simulink model "BD_FUZZY_EMISSIONS"  (Simulink 4.1.1)
settings: Solver=ode1  SolverMode=SingleTasking  StartTime=0.0  StopTime=max(cyc_mph(:,1))  FixedStep=1  MaxStep=1  RelTol=1e-3  AbsTol=1e-3
undefined symbols (not defined in the file): cs_hi_soc, cs_lo_soc, ex_calc, fc_emis, fc_map_spd, fc_max_trq, fc_spd_scale, fc_trq_scale, fc_tstat, fuzzy_target_compute_emissions, mfuzzy_emissions, vc_fc_warm_tmp_frac
libraries: lib_transmission x4, lib_wheel x2, lib_help x2, lib_outputs x1, lib_controls x1, lib_interactive x1, lib_drive_cycle x1, lib_energy_storage x1, lib_exhaust x1, lib_fuel_converter x1, lib_electric_machine x1, lib_power_bus x1
settings Model: LastModifiedBy=ssprik  ModifiedComment=ssprik -- Wed Sep 24 14:56:58 2003 -- Version 1.295  SaveTime=off  SaveOutput=off  LimitDataPoints=off  UnconnectedLineMsg=none  RTWTemplateMakefile=grt_vc.tmf  ExtModeTrigMode=oneshot  ExtModeArmWhenConnect=off
settings Model: ModifiedHistory=|
  | ssprik -- Wed Sep 24 14:56:58 2003 -- Version 1.295
  | 
  | 
  | abrooker -- Tue May 14 11:44:18 2002 -- Version 1.294
  | 
  | 
  | mokeefe -- Thu Apr 18 07:56:06 2002 -- Version 1.293
  | saving the model:
  | o "without the model browser open"
  | o with only top-level screen visible
  | o and with "fit to view" enabled
  | 
  | mokeefe -- Thu Apr 18 07:46:20 2002 -- Version 1.292
  | saving the model:
  | o "without the model browser open"
  | o with only top-level screen visible
  | o and with "fit to view" enabled

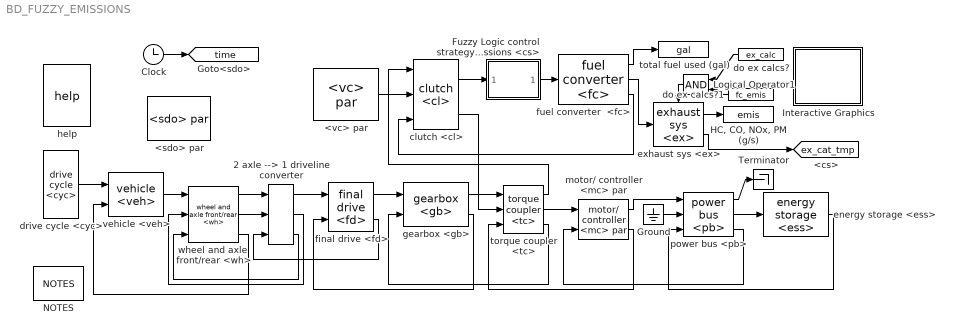
== system BD_FUZZY_EMISSIONS ==
  2 axle --> 1 driveline converter : lib_wheel/2 axle --> 1 driveline converter
      settings: RTWFcnNameOpts=Auto  RTWFileNameOpts=Auto
  <sdo> par : lib_outputs/<sdo> par
  <vc> par : lib_controls/<vc> par
  Clock : Clock
      settings: DisplayTime=off  Decimation=10
  Fuzzy Logic control strategy with Emissions <cs> : Subsystem
      settings: RTWFcnNameOpts=Auto  RTWFileNameOpts=Auto
      mask Display: image(imread('bdi_fuzzy.jpg'))
  Ground : Ground
  "HC, CO, NOx, PM (g/s)" : ToWorkspace  VariableName=emis  SampleTime=0  SaveFormat=Array
  Interactive Graphics : Subsystem  BlockChoice=off
      settings: AttributesFormatString=%<BlockChoice>  TemplateBlock=lib_interactive/Interactive Graphics  MemberBlocks=off,on  RTWFcnNameOpts=Auto  RTWFileNameOpts=Auto
  Logical Operator1 : Logic  Orientation=left  Operator=AND  Inputs=2
  NOTES : lib_help/NOTES
  Terminator : Terminator
  clutch <cl> : lib_transmission/clutch <cl>  slip_spd=vc_launch_spd  maxtrq=max(fc_max_trq)*fc_trq_scale
  do ex calcs? : Constant  Orientation=left  Value=ex_calc
  do ex calcs?1 : Constant  Orientation=left  Value=fc_emis
  drive cycle <cyc> : lib_drive_cycle/drive cycle <cyc>
  energy storage <ess> : lib_energy_storage/energy storage <ess>  AncestorBlock=lib_energy_storage/Subsystem/energy storage <ess>
  exhaust sys <ex> : lib_exhaust/exhaust sys <ex>
  final drive <fd> : lib_transmission/final drive <fd>
  fuel converter  <fc> : lib_fuel_converter/fuel converter  <fc>
  gearbox <gb> : lib_transmission/gearbox <gb>
  help : lib_help/help
  motor/ controller <mc> par : lib_electric_machine/motor// controller <mc> par
  power bus <pb> : lib_power_bus/power bus <pb>
  torque coupler <tc> : lib_transmission/torque coupler <tc>
  total fuel used (gal) : ToWorkspace  VariableName=gal  SampleTime=0  SaveFormat=Array
  vehicle <veh> : lib_vehicle/vehicle <veh>
  wheel and axle  front/rear <wh> : lib_wheel/wheel and axle  front//rear <wh>
  tag scope: ex_cat_tmp=global, time=global
  wires:
  wheel and axle  front/rear <wh>/3 -> vehicle <veh>/2
  final drive <fd>/1 -> gearbox <gb>/1
  drive cycle <cyc>/1 -> vehicle <veh>/1
  clutch <cl>/1 -> Fuzzy Logic control strategy with Emissions <cs>/1("trq and spd req'd into clutch (N*m, rad/s)")
  Fuzzy Logic control strategy with Emissions <cs>/1("trq and spd req'd from engine (N*m, rad/s)") -> fuel converter  <fc>/1
  fuel converter  <fc>/2 -> exhaust sys <ex>/1
  do ex calcs?/1 -> Logical Operator1/1
  fuel converter  <fc>/3 -> clutch <cl>/3
  fuel converter  <fc>/1 -> total fuel used (gal)/1
  exhaust sys <ex>/1 -> "HC, CO, NOx, PM (g/s)"/1
  Logical Operator1/1 -> exhaust sys <ex>/Enable
  do ex calcs?1/1 -> Logical Operator1/2
  Clock/1 -> [time]
  gearbox <gb>/2 -> final drive <fd>/2
  torque coupler <tc>/3 -> gearbox <gb>/2
  torque coupler <tc>/1 -> clutch <cl>/1
  clutch <cl>/2 -> torque coupler <tc>/2
  gearbox <gb>/1 -> torque coupler <tc>/1
  <vc> par/1 -> clutch <cl>/2
  motor/ controller <mc> par/2 -> torque coupler <tc>/3
  motor/ controller <mc> par/1 -> power bus <pb>/1
  Ground/1 -> power bus <pb>/2
  power bus <pb>/3 -> motor/ controller <mc> par/2
  power bus <pb>/2 -> energy storage <ess>/1
  power bus <pb>/1 -> Terminator/1
  energy storage <ess>/1 -> power bus <pb>/3
  torque coupler <tc>/2 -> motor/ controller <mc> par/1
  exhaust sys <ex>/2 -> [ex_cat_tmp]
  vehicle <veh>/1 -> wheel and axle  front/rear <wh>/1
  wheel and axle  front/rear <wh>/1 -> 2 axle --> 1 driveline converter/1
  wheel and axle  front/rear <wh>/2 -> 2 axle --> 1 driveline converter/2
  2 axle --> 1 driveline converter/1 -> final drive <fd>/1
  2 axle --> 1 driveline converter/2 -> wheel and axle  front/rear <wh>/2
  2 axle --> 1 driveline converter/3 -> wheel and axle  front/rear <wh>/3
  final drive <fd>/2 -> 2 axle --> 1 driveline converter/3

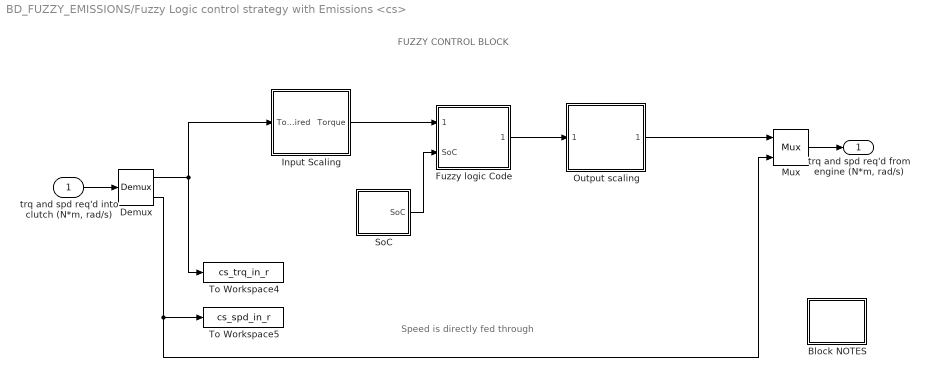
== system BD_FUZZY_EMISSIONS/Fuzzy Logic control strategy with Emissions <cs> ==
  note: FUZZY CONTROL BLOCK
  note: Speed is directly fed through
  "trq and spd req'd into clutch (N*m, rad/s)" : Inport  Port=1  LatchInput=off
  Block NOTES : Subsystem
      settings: RTWFcnNameOpts=Auto  RTWFileNameOpts=Auto
      mask Display: disp('Block\nNOTES')
  Demux : Demux  Outputs=2  BusSelectionMode=off
  Fuzzy logic Code : Subsystem
      settings: RTWFcnNameOpts=Auto  RTWFileNameOpts=Auto
  Input Scaling : Subsystem
      settings: RTWFcnNameOpts=Auto  RTWFileNameOpts=Auto
  Mux : Mux  Inputs=2
      settings: DisplayOption=none
  Output scaling : Subsystem
      settings: RTWFcnNameOpts=Auto  RTWFileNameOpts=Auto
  "SoC " : Subsystem
      settings: RTWFcnNameOpts=Auto  RTWFileNameOpts=Auto
  To Workspace4 : ToWorkspace  VariableName=cs_trq_in_r  SampleTime=-1  SaveFormat=Array
  To Workspace5 : ToWorkspace  VariableName=cs_spd_in_r  SampleTime=-1  SaveFormat=Array
  "trq and spd req'd from engine (N*m, rad/s)" : Outport  Port=1
  wires:
  Fuzzy logic Code/1(delta  alpha) -> Output scaling/1("delta alpha ")
  Input Scaling/1(Torque) -> Fuzzy logic Code/1(Torque)
  "trq and spd req'd into clutch (N*m, rad/s)"/1 -> Demux/1
  Demux/2 -> To Workspace5/1, Mux/2
  Demux/1 -> To Workspace4/1, Input Scaling/1(Torque required)
  Mux/1 -> "trq and spd req'd from engine (N*m, rad/s)"/1
  "SoC "/1(SoC) -> Fuzzy logic Code/2(SoC)
  Output scaling/1(ICE Torque command) -> Mux/1

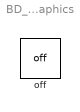
== system BD_FUZZY_EMISSIONS/Interactive Graphics ==
  off : lib_interactive/off  Tag=Altia_off  Orientation=up

== system BD_FUZZY_EMISSIONS/Fuzzy Logic control strategy with Emissions <cs>/Block NOTES ==
  note: The Fuzzy Control Block takes in the torque and speed requested by the clutch (sink) and calculates
      | the torque split between the ICE and the Motor. The fuzzy logic algorithm sets a base (optimal)
      | operating point of the ICE and modifies the actual operating point about the optimal, based on
      | the actual torque request and the battery State of Charge (SOC). Finally, a torque request is sent to the
      | ICE and the motor buffers the remaining torque (positive or negative).

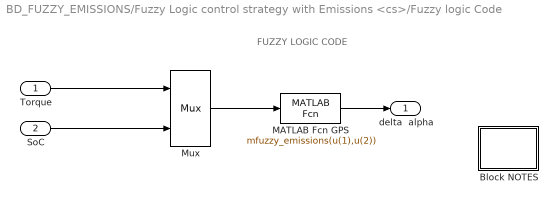
== system BD_FUZZY_EMISSIONS/Fuzzy Logic control strategy with Emissions <cs>/Fuzzy logic Code ==
  note: FUZZY LOGIC CODE
  Torque : Inport  Port=1  LatchInput=off
  SoC : Inport  Port=2  LatchInput=off
  Block NOTES : Subsystem
      settings: RTWFcnNameOpts=Auto  RTWFileNameOpts=Auto
      mask Display: disp('Block\nNOTES')
  "MATLAB Fcn GPS " : MATLABFcn  MATLABFcn=mfuzzy_emissions(u(1),u(2))  OutputDimensions=1  OutputSignalType=auto  Output1D=on
  Mux : Mux  Inputs=2
      settings: DisplayOption=none
  delta  alpha : Outport  Port=1
  wires:
  Mux/1 -> "MATLAB Fcn GPS "/1
  Torque/1 -> Mux/1
  "MATLAB Fcn GPS "/1 -> delta  alpha/1
  SoC/1 -> Mux/2

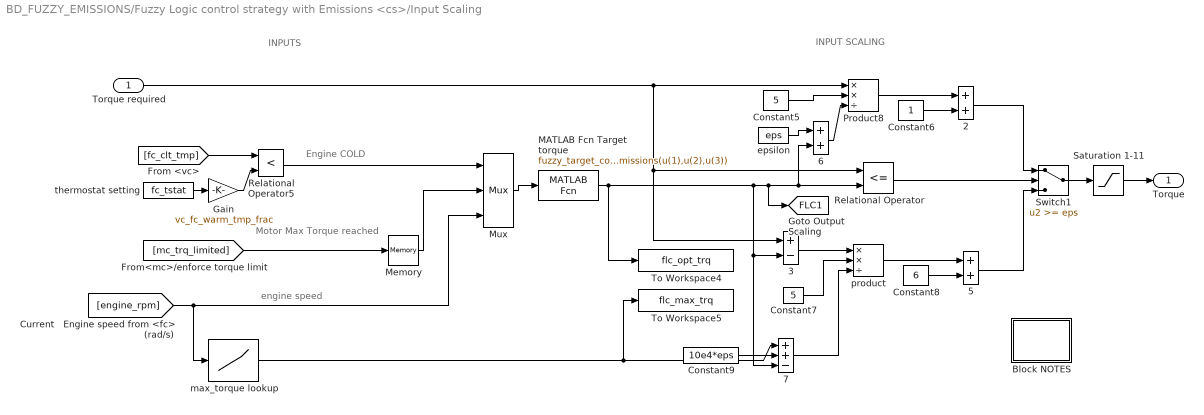
== system BD_FUZZY_EMISSIONS/Fuzzy Logic control strategy with Emissions <cs>/Input Scaling ==
  note: INPUTS
  note: INPUT SCALING
  note: Engine COLD
  note: Motor Max
      | Torque reached
  note: engine speed
  Torque required : Inport  Port=1  LatchInput=off
  " 2" : Sum  Inputs=++  SaturateOnIntegerOverflow=on
  " 3" : Sum  Inputs=+-  SaturateOnIntegerOverflow=on
  " 5" : Sum  Inputs=++  SaturateOnIntegerOverflow=on
  " 6" : Sum  Inputs=++  SaturateOnIntegerOverflow=on
  " 7" : Sum  Inputs=++-  SaturateOnIntegerOverflow=on
  Block NOTES : Subsystem
      settings: RTWFcnNameOpts=Auto  RTWFileNameOpts=Auto
      mask Display: disp('Block\nNOTES')
  Constant5 : Constant  Value=5
  Constant6 : Constant  Value=1
  Constant7 : Constant  Value=5
  Constant8 : Constant  Value=6
  Constant9 : Constant  Value=10e4*eps
  Gain : Gain  Gain=vc_fc_warm_tmp_frac  Multiplication=Element-wise(K.*u)  SaturateOnIntegerOverflow=on
  MATLAB Fcn Target torque : MATLABFcn  MATLABFcn=fuzzy_target_compute_emissions(u(1),u(2),u(3))  OutputDimensions=1  OutputSignalType=auto  Output1D=on
  Memory : Memory  X0=0  InheritSampleTime=off
      settings: RTWStateStorageClass=Auto
  Mux : Mux  Inputs=3
      settings: DisplayOption=none
  Product8 : Product  Inputs=**/  Multiplication=Element-wise(.*)  SaturateOnIntegerOverflow=on
  Relational Operator : RelationalOperator  Operator=<=
  Relational Operator5 : RelationalOperator  Operator=<
  "Saturation 1-11 " : Saturate  UpperLimit=11  LowerLimit=1  LinearizeAsGain=on
  Switch1 : Switch  Threshold=eps
  To Workspace4 : ToWorkspace  VariableName=flc_opt_trq  SampleTime=-1  SaveFormat=Array
  To Workspace5 : ToWorkspace  VariableName=flc_max_trq  SampleTime=-1  SaveFormat=Array
  epsilon : Constant  Value=eps
  max_torque lookup : Lookup  InputValues=fc_map_spd*fc_spd_scale  OutputValues=fc_max_trq*fc_trq_scale
  product : Product  Inputs=**/  Multiplication=Element-wise(.*)  SaturateOnIntegerOverflow=on
  thermostat setting : Constant  Value=fc_tstat
  Torque : Outport  Port=1
  tag scope: FLC1=global
  wires:
  Switch1/1 -> "Saturation 1-11 "/1
  " 7"/1 -> product/3
  " 6"/1 -> Product8/3
  epsilon/1 -> " 6"/1
  Constant9/1 -> " 7"/2
  Constant5/1 -> Product8/2
  "Saturation 1-11 "/1 -> Torque/1
  " 5"/1 -> Switch1/3
  product/1 -> " 5"/1
  Constant8/1 -> " 5"/2
  Constant7/1 -> product/2
  " 3"/1 -> product/1
  " 2"/1 -> Switch1/1
  Constant6/1 -> " 2"/2
  Product8/1 -> " 2"/1
  Relational Operator/1 -> Switch1/2
  MATLAB Fcn Target torque/1 -> To Workspace4/1, " 7"/3, " 3"/2, " 6"/2, Relational Operator/2, [FLC1]
  [engine_rpm] -> max_torque lookup/1, Mux/3
  Mux/1 -> MATLAB Fcn Target torque/1
  max_torque lookup/1 -> " 7"/1, To Workspace5/1
  Torque required/1 -> " 3"/1, Relational Operator/1, Product8/1
  [mc_trq_limited] -> Memory/1
  thermostat setting/1 -> Gain/1
  Gain/1 -> Relational Operator5/2
  [fc_clt_tmp] -> Relational Operator5/1
  Relational Operator5/1 -> Mux/1
  Memory/1 -> Mux/2

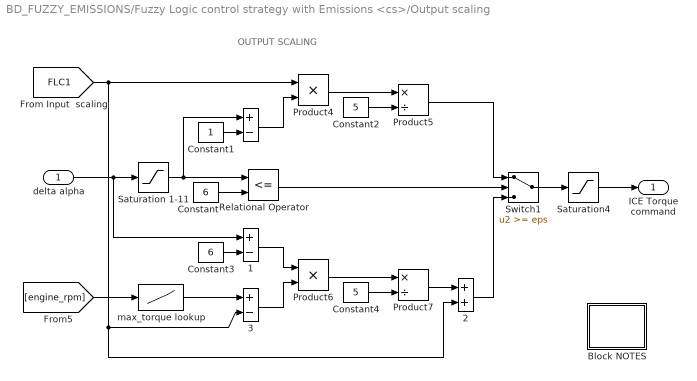
== system BD_FUZZY_EMISSIONS/Fuzzy Logic control strategy with Emissions <cs>/Output scaling ==
  note: OUTPUT SCALING
  "delta alpha " : Inport  Port=1  LatchInput=off
  " " : Sum  Inputs=+-  SaturateOnIntegerOverflow=on
  " 1" : Sum  Inputs=+-  SaturateOnIntegerOverflow=on
  " 2" : Sum  Inputs=++  SaturateOnIntegerOverflow=on
  " 3" : Sum  Inputs=+-  SaturateOnIntegerOverflow=on
  Block NOTES : Subsystem
      settings: RTWFcnNameOpts=Auto  RTWFileNameOpts=Auto
      mask Display: disp('Block\nNOTES')
  Constant : Constant  Value=6
  Constant1 : Constant  Value=1
  Constant2 : Constant  Value=5
  Constant3 : Constant  Value=6
  Constant4 : Constant  Value=5
  Product4 : Product  Inputs=2  Multiplication=Element-wise(.*)  SaturateOnIntegerOverflow=on
  Product5 : Product  Inputs=*/  Multiplication=Element-wise(.*)  SaturateOnIntegerOverflow=on
  Product6 : Product  Inputs=2  Multiplication=Element-wise(.*)  SaturateOnIntegerOverflow=on
  Product7 : Product  Inputs=*/  Multiplication=Element-wise(.*)  SaturateOnIntegerOverflow=on
  Relational Operator : RelationalOperator  Operator=<=
  Saturation 1-11 : Saturate  UpperLimit=11  LowerLimit=1  LinearizeAsGain=on
  Saturation4 : Saturate  UpperLimit=max(fc_max_trq*fc_trq_scale)  LowerLimit=0  LinearizeAsGain=on
  Switch1 : Switch  Threshold=eps
  max_torque lookup : Lookup  InputValues=fc_map_spd*fc_spd_scale  OutputValues=fc_max_trq*fc_trq_scale
  ICE Torque command : Outport  Port=1
  wires:
  max_torque lookup/1 -> " 3"/1
  [engine_rpm] -> max_torque lookup/1
  Saturation4/1 -> ICE Torque command/1
  Switch1/1 -> Saturation4/1
  Product7/1 -> " 2"/1
  " 2"/1 -> Switch1/3
  Relational Operator/1 -> Switch1/2
  Product5/1 -> Switch1/1
  Constant4/1 -> Product7/2
  Product6/1 -> Product7/1
  " 3"/1 -> Product6/2
  " 1"/1 -> Product6/1
  Constant3/1 -> " 1"/2
  "delta alpha "/1 -> Saturation 1-11/1, " 1"/1
  [FLC1] -> " 3"/2, " 2"/2, Product4/1
  Constant2/1 -> Product5/2
  Product4/1 -> Product5/1
  " "/1 -> Product4/2
  Saturation 1-11/1 -> " "/1, Relational Operator/1
  Constant1/1 -> " "/2
  Constant/1 -> Relational Operator/2

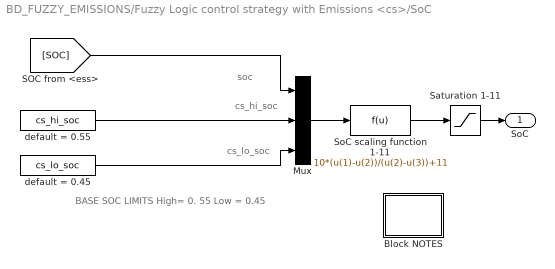
== system BD_FUZZY_EMISSIONS/Fuzzy Logic control strategy with Emissions <cs>/SoC  ==
  note: soc
  note: cs_hi_soc
  note: cs_lo_soc
  note: BASE SOC LIMITS
      | High= 0. 55
      | Low  = 0.45
  Block NOTES : Subsystem
      settings: RTWFcnNameOpts=Auto  RTWFileNameOpts=Auto
      mask Display: disp('Block\nNOTES')
  Mux : Mux  Inputs=3
  Saturation 1-11 : Saturate  UpperLimit=11  LowerLimit=1  LinearizeAsGain=on
  SoC scaling function 1-11 : Fcn  Expr=10*(u(1)-u(2))/(u(2)-u(3))+11
  default = 0.45 : Constant  Value=cs_lo_soc
  default = 0.55 : Constant  Value=cs_hi_soc
  SoC : Outport  Port=1
  wires:
  Mux/1 -> SoC scaling function 1-11/1
  [SOC] -> Mux/1
  default = 0.55/1 -> Mux/2
  default = 0.45/1 -> Mux/3
  SoC scaling function 1-11/1 -> Saturation 1-11/1
  Saturation 1-11/1 -> SoC/1

== system BD_FUZZY_EMISSIONS/Fuzzy Logic control strategy with Emissions <cs>/Fuzzy logic Code/Block NOTES ==
  note: This block calls the Fuzzy Controller through the Matlab-Function module.
      | The Fuzzy Control algorithm is written in MATLAB script. This makes it easy
      | for the user to edit the fuzzy algorithm and make changes.
      |
      | For more information on Matlab-functions, please refer to the MATLAB help files.

== system BD_FUZZY_EMISSIONS/Fuzzy Logic control strategy with Emissions <cs>/Input Scaling/Block NOTES ==
  note: In this block, inputs to the Fuzzy Logic controller are computed. The Current torque demand on the ICE
      | and the SoC are input as 2 scaled variables to the fuzzy controller. Both inputs are scaled from 1 to 11.
      |
      | For SoC, a value of cs_lo_soc would correspond to 1 and a value of cs_hi_soc would correspond to 11,
      | linearly interpolating between them.
      |
      | For the ICE Torque, any torque demand less than the target ICE torque would scale from 1 to 6. Any torque
      | demand greater than the target ICE torque would scale from 6 to 11 (the 2 being piecewise linear).
  note: INPUT SCALING
  note: TARGET TORQUE COMPUTATION
  note: The target (optimal) torque for a particular speed requested from the ICE is calculated using a weighted average of
      | the efficiency and emissions data for a particular speed in consideration.
      |
      | The calculation of the target torque involves calculating the minimum of a cost function. The competing quantities
      | of the cost function include the emissions and fuel economy for all torques at that speed, weighed by their
      | respective weights.
      |
      | The relative importance for the competing quantities (weights) are changed during the simulation,
      | to reflect changes in driving conditions. For example, during a cold start, emissions are given higher priority. Also,
      | if the electric motor has been reaching it's maximum assist capability in the wake of the torque request not being met,
      | then emissions are sacrificed for higher torque from the ICE.

== system BD_FUZZY_EMISSIONS/Fuzzy Logic control strategy with Emissions <cs>/Output scaling/Block NOTES ==
  note: OUTPUT SCALING
      | This bock scales the outputs of the controller to match the size of the components.
      | The scaling affects the way control signal is fed into the actuators. The scaling is done based
      | on the membership functions of the Fuzzy Control block.
      |
      | Here:
      |  DELTA ALPHA is scaled from 1 to 11, 1 representing zero torque, 6 representing target Torque
      | and 11 representing Max ICE torque. (the 2 regions being piecewise linear).

== system BD_FUZZY_EMISSIONS/Fuzzy Logic control strategy with Emissions <cs>/SoC /Block NOTES ==
  note: This block scales the battery SOC so as to feed it into the Fuzzy controller.
      | 1 represents the lower limit of allowable battery SOC while 11 represents the higher
      | limit of allowable battery SOC.
